simulink model "Lab3_Crazyflie_Task2_3"  (R2020a)
settings: Solver=FixedStepAuto  StartTime=0.0  StopTime=inf  MaxStep=0.1  RelTol=1e-3  EnableMultiTasking=on
PreLoadFcn:
  | % load parameters of the default quadrotor
  | disp('Quadrotor parameters loaded by PreLoadFcn')
  | mdl_quadrotor
values from neighbouring files (symbols this model uses):
  xx = via(:,1)    [Lab3_trajectories.m]
  yawyaw = 0 .* via(:,1)    [Lab3_trajectories.m]
  yy = via(:,2)    [Lab3_trajectories.m]
  zz = via(:,3) + 1    [Lab3_trajectories.m]
undefined symbols (not defined in the file or in its folder): angdiff, Pitch, Roll, rot2, Thrust, YawRate
libraries: simulink x7, robotlib x3
settings Model: Creator=corkep  LastModifiedBy=Pablo
settings DataIOCC: LimitDataPoints=on  ReturnWorkspaceOutputs=off
settings OptimizationCC: EnhancedBackFolding=on  PassReuseOutputArgsAs=Individual arguments  ExpressionDepthLimit=2147483647  ZeroExternalMemoryAtStartup=off  ZeroInternalMemoryAtStartup=off  MaxStackSize=64  OptimizeBlockOrder=speed  DifferentSizesBufferReuse=on  OptimizationCustomize=off  EfficientTunableParamExpr=on
settings DebuggingCC: UnderspecifiedInitializationDetection=Classic  MergeDetectMultiDrivingBlocksExec=none  SolverPrmCheckMsg=warning  ParameterTunabilityLossMsg=error  AllowSymbolicDim=off  StateNameClashWarn=warning  SFUnexpectedBacktrackingDiag=warning  SFNoUnconditionalDefaultTransitionDiag=warning  SFExecutionAtInitializationDiag=none  ArithmeticOperatorsInVariantConditions=warning
settings HardwareCC: ProdBitPerPointer=32  ProdBitPerSizeT=32  ProdBitPerPtrDiffT=32  ProdLargestAtomicFloat=None  ProdIntDivRoundTo=Undefined  ProdEndianess=Unspecified  ProdWordSize=32  ProdHWDeviceType=Generic->Unspecified (assume 32-bit Generic)  UseEmbeddedCoderFeatures=off
settings ModelReferenceCC: PropagateSignalLabelsOutOfModel=off
settings SFSimCC: SimUseLocalCustomCode=off  MATLABDynamicMemAlloc=off  CustomCodeUndefinedFunction=UseInterfaceOnly
settings RTWCC: SystemTargetFile=ert.tlc  HardwareBoard=Robot Operating System (ROS)  TemplateMakefile=ert_default_tmf  RTWUseLocalCustomCode=off  Toolchain=Catkin  TargetLang=C++
settings CodeAppCC: ForceParamTrailComments=on  IgnoreCustomStorageClasses=off  OperatorAnnotations=on  SimulinkDataObjDesc=on  SFDataObjDesc=on  InsertBlockDesc=on
settings ERTTargetCC: SupportNonInlinedSFcns=on
settings ConfigComp: CovMetricSettings=dw  CovHtmlReporting=on  CovSaveCumulativeToWorkspaceVar=on  CovSaveSingleToWorkspaceVar=on  CovExternalEMLEnable=off  CovSFcnEnable=off

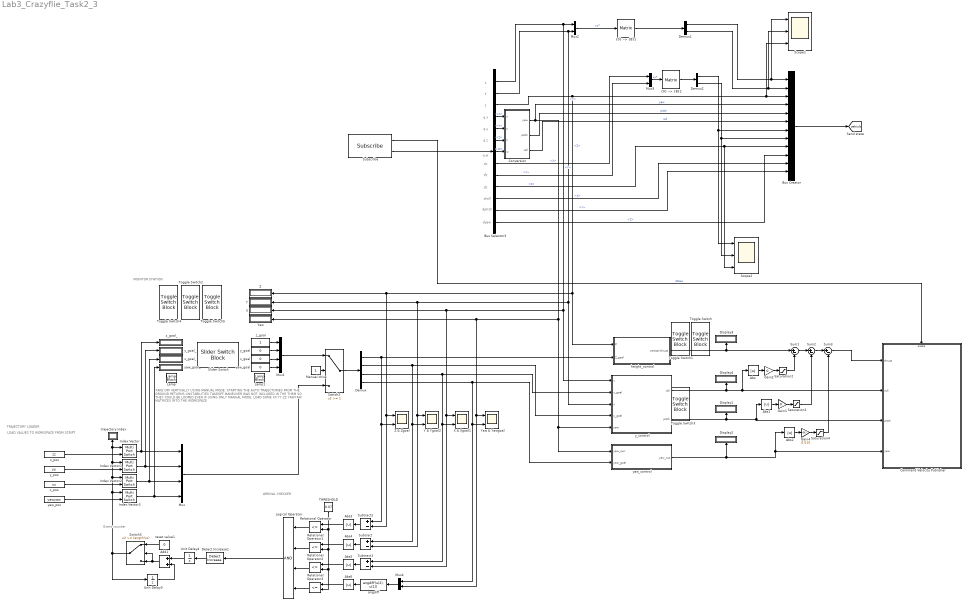
== system Lab3_Crazyflie_Task2_3 ==
  note: TAKE OFF VERTICALLY USING MANUAL MODE:
      | STARTING THE AUTO TRAJECTORIES FROM THE GROUND RETURNS UNSTABILITIES
      | TAKEOFF MANEUVER WAS NOT INCLUDED IN THE THEM SO THEY COULD BE LOOPED
      | EVEN IF USING ONLY MANUAL MODE, LOAD SOME XX YY ZZ YAWYAW MATRICES INTO THE WORKSPACE
  note: MONITOR STATION
  note: ARRIVAL CHECKER
  note: TRAJECTORY LOADER
  note: dyaw
  note: dpitch
  note: droll
  note: dz
  note: dy
  note: dx
  note: x
  note: y
  note: z
  note: q.x
  note: q.y
  note: q.z
  note: q.w
  note: LOAD VALUES TO WORKSPACE
      | FROM SCRIPT
  note: Event counter
  Abs{,1..6} (7 alike) : Abs
  Add1 : Sum
  Bus Creator : BusCreator  Inputs=12
  Bus Selector3 : BusSelector  OutputSignals=Pose.Pose.Position.X,Pose.Pose.Position.Y,Pose.Pose.Position.Z,Pose.Pose.Orientation.X,Pose.Pose.Orientation.Y,Pose.Pose.Orientation.Z,Pose.Pose.Orientation.W,Twist.Twist.Linear.X,Twist.Twist.Linear.Y,Twist.Twist.Linear.Z,Twist.Twist.Angular.X,Twist.Twist.Angular.Y,Twist.Twist.Angular.Z
  Command Velocity Publisher : Subsystem
  Conversion : MATLAB Function  TreatAsAtomicUnit=on
  Demux : Demux
  Demux1 : Demux  Outputs=2
  Demux2 : Demux  Outputs=2
  Detect Increase1 : simulink/Logic and Bit Operations/Detect Increase  vinit=0.0  OutDataTypeStr=boolean
  Display{1..4} (4 alike) : Display
  Gain1 : Gain  Gain=0
  Gain2 : Gain  Gain=0
  Gain4 : Gain  Gain=0.015
  Index Vector{,1..3} (4 alike) : MultiPortSwitch  DataPortOrder=Zero-based contiguous  Inputs=1  zeroidx=on
  Lamp : LampBlock
  Lamp1 : LampBlock
  Logical Operator : Logic  Inputs=4  AllPortsSameDT=off  OutDataTypeStr=boolean
  Manual drive : Constant
  Mux : Mux
  Mux1 : Mux
  Mux2 : Mux  Inputs=2
  Mux3 : Mux  Inputs=2
  Mux4 : Mux  Inputs=2
  Relational Operator{,1..3} (4 alike) : RelationalOperator  Operator=<=  OutDataTypeStr=boolean  RndMeth=Simplest
  Saturation1 : Saturate  LowerLimit=0
  Saturation2 : Saturate  LowerLimit=0
  Saturation4 : Saturate  LowerLimit=0
  Scope1 : Scope  NumInputPorts=3
  Scope2 : Scope  NumInputPorts=3
  Slider Switch : SliderSwitchBlock
      settings: Values={{'Auto', 'Manual'}, [0 1]}
  Subscribe : robotlib/Subscribe  topicSource=Select from ROS network  topic=/crazyflie2/ground_truth/odometry  messageType=nav_msgs/Odometry  sampleTime=-1  messageQueueLength=51
  Subtract : Sum  Inputs=+-
  Subtract1 : Sum  Inputs=+-
  Subtract2 : Sum  Inputs=+-
  Sum1 : Sum  Inputs=|+-
  Sum2 : Sum  Inputs=|+-
  Sum3 : Sum  Inputs=|+-
  Switch2 : Switch  Threshold=1
  Switch3 : Switch  Threshold=length(xx)
  THRESHOLD : Constant  Value=0.07
  Toggle Switch{,1..5} (6 alike) : ToggleSwitchBlock
      settings: Values={{'Off', 'On'}, [0 1]}
  Unit Delay3 : UnitDelay  SampleTime=-1  HasFrameUpgradeWarning=on
  Unit Delay4 : UnitDelay  SampleTime=-1  HasFrameUpgradeWarning=on
  X : Display
  X & Xgoal1 : Scope  NumInputPorts=2
  Y : Display
  Y & Ygoal2 : Scope  NumInputPorts=2
  Yaw : Display
  Yaw & Yawgoal : Scope  NumInputPorts=2
  Z : Display
  Z & Zgoal : Scope  NumInputPorts=2
  angdiff : MATLABFcn  MATLABFcn=angdiff(u(2), u(1))  OutputDimensions=1  Output1D=off
  height_control : Subsystem
  reset value1 : Constant  Value=0  VectorParams1D=off
  trajectory index : Display
  x_goal : Constant  Value=0
  x_goal_ : Display
  x_pos : Constant  Value=xx  VectorParams1D=off
  y_control : Subsystem
  y_goal : Constant  Value=0
  y_goal_ : Display
  y_pos : Constant  Value=yy  VectorParams1D=off
  yaw_control : Subsystem
  yaw_goal : Constant  Value=0
  yaw_goal_ : Display
  yaw_pos : Constant  Value=yawyaw  VectorParams1D=off
  z_goal : Constant
  z_goal_ : Display
  z_pos : Constant  Value=zz  VectorParams1D=off
  "{0} --> {B}1" : Product  Inputs=1  Multiplication=Matrix(*)  RndMeth=Zero
  "{0} --> {B}2" : Product  Inputs=1  Multiplication=Matrix(*)  RndMeth=Zero
  tag scope: vehicle=global
  wires:
  Bus Selector3/11 -> Bus Creator/11  "<X>"
  Bus Selector3/13 -> Bus Creator/10  "<Z>"
  Conversion/1(yaw) -> Bus Creator/4, yaw_control/1(yaw_curr), y_control/5(yaw), Yaw/1, Mux4/2, Yaw & Yawgoal/1  "yaw"
  Bus Selector3/10 -> Bus Creator/9, Scope2/3  "<Z>"
  Bus Selector3/9 -> Mux3/2  "<Y>"
  Bus Selector3/8 -> Mux3/1  "<X>"
  Conversion/2(pitch) -> Bus Creator/5  "pitch"
  Bus Selector3/3 -> Scope1/3, Bus Creator/3, height_control/1(Z), Subtract2/2, Z & Zgoal/1, Z/1  "<Z>"
  Bus Creator/1 -> [vehicle]
  Bus Selector3/12 -> Bus Creator/12  "<Y>"
  Conversion/3(roll) -> Bus Creator/6  "roll"
  Subscribe/2 -> Bus Selector3/1
  Bus Selector3/4 -> Conversion/1(x)  "<X>"
  Bus Selector3/5 -> Conversion/2(y)  "<Y>"
  Bus Selector3/6 -> Conversion/3(z)  "<Z>"
  Bus Selector3/7 -> Conversion/4(w)  "<W>"
  Subscribe/1 -> Command Velocity Publisher/Enable  "IsNew"
  Mux2/1 -> "{0} --> {B}1"/1  "xy*"
  "{0} --> {B}1"/1 -> Demux1/1
  "{0} --> {B}2"/1 -> Demux2/1
  Mux3/1 -> "{0} --> {B}2"/1  "xy*"
  Demux1/1 -> Bus Creator/1, Scope1/1
  Demux1/2 -> Bus Creator/2, Scope1/2
  Bus Selector3/1 -> Mux2/1, y_control/1(x), Subtract1/2, X & Xgoal1/1, X/1  "<X>"
  Demux2/1 -> Bus Creator/7, Scope2/1
  Demux2/2 -> Bus Creator/8, Scope2/2
  height_control/1(vertical thrust) -> Display3/1, Sum1/1
  Demux/1 -> Subtract2/1, Z & Zgoal/2, height_control/2(Z_goal)
  Bus Selector3/2 -> y_control/3(y), Subtract/2, Y & Ygoal2/1, Y/1, Mux2/2  "<Y>"
  Demux/3 -> X & Xgoal1/2, Subtract1/1, y_control/2(x_goal)
  Demux/4 -> Mux4/1, Yaw & Yawgoal/2, yaw_control/2(yaw_goal)
  Demux/2 -> Subtract/1, Y & Ygoal2/2, y_control/4(y_goal)
  Sum1/1 -> Sum2/1
  Sum2/1 -> Sum3/1
  Gain2/1 -> Saturation2/1
  Abs/1 -> Gain2/1
  Abs1/1 -> Gain1/1
  Gain1/1 -> Saturation1/1
  Saturation2/1 -> Sum1/2
  Saturation1/1 -> Sum2/2
  Abs2/1 -> Gain4/1
  Gain4/1 -> Saturation4/1
  Saturation4/1 -> Sum3/2
  z_pos/1 -> Index Vector/2
  y_pos/1 -> Index Vector1/2
  Index Vector2/1 -> Mux/3, x_goal_/1
  x_pos/1 -> Index Vector2/2
  Index Vector/1 -> Mux/1, z_goal_/1
  Index Vector1/1 -> Mux/2, y_goal_/1
  Switch3/1 -> Unit Delay3/1, trajectory index/1, Index Vector/1, Index Vector1/1, Index Vector2/1, Index Vector3/1
  yaw_pos/1 -> Index Vector3/2
  Index Vector3/1 -> yaw_goal_/1, Mux/4
  Mux/1 -> Switch2/3
  z_goal/1 -> Mux1/1
  y_goal/1 -> Mux1/2
  x_goal/1 -> Mux1/3
  yaw_goal/1 -> Mux1/4
  Mux1/1 -> Switch2/1
  Switch2/1 -> Demux/1
  Manual drive/1 -> Switch2/2
  Add1/1 -> Switch3/2, Switch3/3
  Unit Delay3/1 -> Add1/2
  reset value1/1 -> Switch3/1
  Detect Increase1/1 -> Unit Delay4/1
  Unit Delay4/1 -> Add1/1
  Logical Operator/1 -> Detect Increase1/1
  Mux4/1 -> angdiff/1
  Subtract2/1 -> Abs3/1
  Subtract/1 -> Abs4/1
  Subtract1/1 -> Abs5/1
  angdiff/1 -> Abs6/1
  Abs3/1 -> Relational Operator/1
  Abs4/1 -> Relational Operator1/1
  Abs5/1 -> Relational Operator2/1
  Abs6/1 -> Relational Operator3/1
  THRESHOLD/1 -> Relational Operator/2, Relational Operator1/2, Relational Operator2/2, Relational Operator3/2
  Relational Operator/1 -> Logical Operator/1
  Relational Operator1/1 -> Logical Operator/2
  Relational Operator2/1 -> Logical Operator/3
  Relational Operator3/1 -> Logical Operator/4
  Sum3/1 -> Command Velocity Publisher/1(thrust)
  y_control/1(roll) -> Display4/1, Abs/1, Command Velocity Publisher/2(roll)
  y_control/2(pitch) -> Display1/1, Abs1/1, Command Velocity Publisher/3(pitch)
  yaw_control/1(yaw_out) -> Display2/1, Command Velocity Publisher/4(yaw), Abs2/1

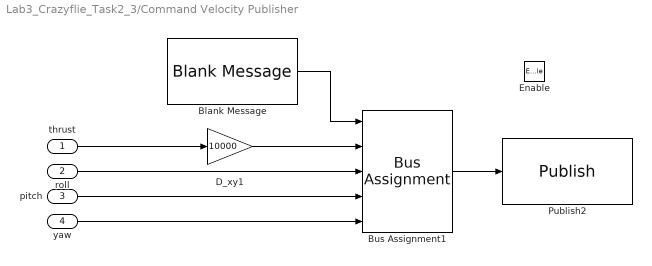
== system Lab3_Crazyflie_Task2_3/Command Velocity Publisher ==
  thrust : Inport
  roll : Inport  Port=2
  pitch : Inport  Port=3
  yaw : Inport  Port=4
  Enable : EnablePort
  Blank Message : robotlib/Blank Message  messageClass=Message  entityType=mav_msgs/RollPitchYawrateThrustCrazyflie  messageType=mav_msgs/RollPitchYawrateThrustCrazyflie  SampleTime=inf
  Bus Assignment1 : BusAssignment  DialogController=Simulink.DDGSource_BusAssignment  AssignedSignals=Thrust,Roll,Pitch,YawRate
  D_xy1 : Gain  Gain=10000
  Publish2 : robotlib/Publish  topicSource=Select from ROS network  topic=/crazyflie2/command/roll_pitch_yawrate_thrust  messageType=mav_msgs/RollPitchYawrateThrustCrazyflie  messageQueueLength=105
  wires:
  Blank Message/1 -> Bus Assignment1/1
  Bus Assignment1/1 -> Publish2/1
  thrust/1 -> D_xy1/1
  roll/1 -> Bus Assignment1/3
  pitch/1 -> Bus Assignment1/4
  yaw/1 -> Bus Assignment1/5
  D_xy1/1 -> Bus Assignment1/2

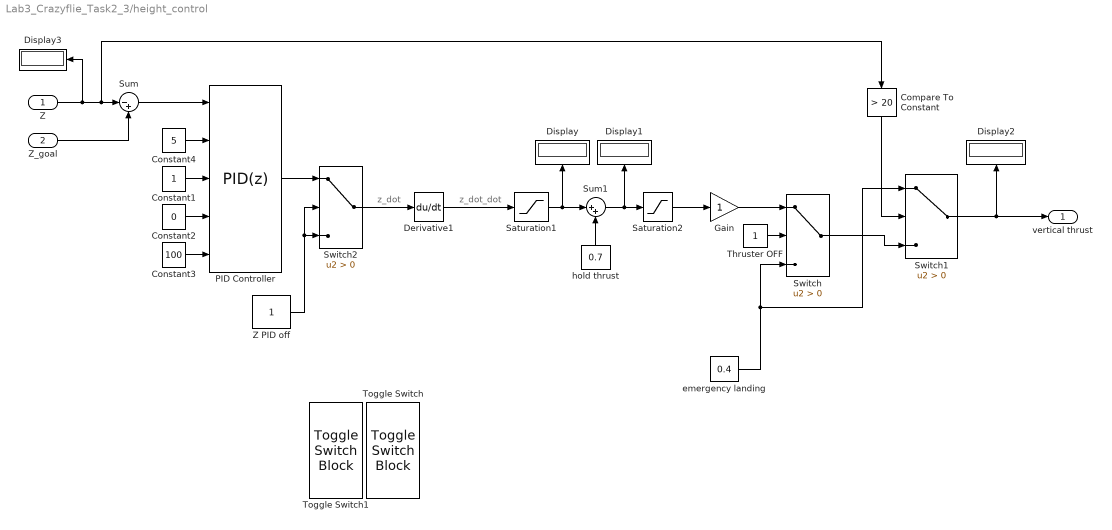
== system Lab3_Crazyflie_Task2_3/height_control ==
  note: z_dot
  note: z_dot_dot
  Z : Inport
  Z_goal : Inport  Port=2
  Compare To Constant : simulink/Logic and Bit Operations/Compare To Constant  relop=>  const=20  OutDataTypeStr=boolean
  Constant1 : Constant
  Constant2 : Constant  Value=0
  Constant3 : Constant  Value=100
  Constant4 : Constant  Value=5
  Derivative1 : Derivative
  Display{,1..3} (4 alike) : Display
  Gain : Gain
  PID Controller : simulink/Continuous/PID Controller  Controller=PID  Form=Parallel  TimeDomain=Discrete-time  UseExternalTs=off  SampleTime=-1  IntegratorMethod=Forward Euler  FilterMethod=Forward Euler  ControllerParametersSource=external  P=1  I=0  D=0  UseFilter=on  N=1000  TunerSelectOption=Transfer Function Based (PID Tuner App)  InitialConditionSource=internal  InitialConditionForIntegrator=0  InitialConditionForFilter=0  DifferentiatorICPrevScaledInput=0  ExternalReset=none  TrackingMode=off  Kt=1  LimitOutput=off  UpperSaturationLimit=inf  LowerSaturationLimit=-inf  LinearizeAsGain=on  AntiWindupMode=none  Kb=1  POutMin=[]  POutMax=[]  IOutMin=[]  IOutMax=[]  DOutMin=[]  DOutMax=[]  NOutMin=[]  NOutMax=[]  SumOutMin=[]  SumOutMax=[]  SaturationOutMin=[]  SaturationOutMax=[]  PParamMin=[]  PParamMax=[]  IParamMin=[]  IParamMax=[]  DParamMin=[]  DParamMax=[]  NParamMin=[]  NParamMax=[]  KbParamMin=[]  KbParamMax=[]  KtParamMin=[]  KtParamMax=[]  KbOutMin=[]  KbOutMax=[]  KtOutMin=[]  KtOutMax=[]  IntegratorOutMin=[]  IntegratorOutMax=[]  FilterOutMin=[]  FilterOutMax=[]  SumI1OutMin=[]  SumI1OutMax=[]  SumI2OutMin=[]  SumI2OutMax=[]  SumI3OutMin=[]  SumI3OutMax=[]  SumI4OutMin=[]  SumI4OutMax=[]  SumDOutMin=[]  SumDOutMax=[]  DifferentiatorOutMin=[]  DifferentiatorOutMax=[]  FilterDiffOutCoefMin=[]  FilterDiffOutCoefMax=[]  ReciprocalOutMin=[]  ReciprocalOutMax=[]  SumDenOutMin=[]  SumDenOutMax=[]  SumNumOutMin=[]  SumNumOutMax=[]  DivideOutMin=[]  DivideOutMax=[]  UdiffTsProdOutMin=[]  UdiffTsProdOutMax=[]  NTsProdOutMin=[]  NTsProdOutMax=[]  UintegralTsProdOutMin=[]  UintegralTsProdOutMax=[]  UngainTsProdOutMin=[]  UngainTsProdOutMax=[]  IntegratorContinuousStateAttributes=''  IntegratorStateMustResolveToSignalObject=off  IntegratorRTWStateStorageClass=Auto  FilterContinuousStateAttributes=''  FilterStateMustResolveToSignalObject=off  FilterRTWStateStorageClass=Auto  ParallelPVariant=ExternalParameters  IdealPVariant=Disabled  IVariant=ExternalParameters  DVariant=ExternalParameters  IntegratorVariant=Discrete  SatVariant=Disabled  AWVariant=Passthrough  PCopyVariant=Disabled  TRVariant=Disabled  FdbkBlocksVariant=Forward  IdealPFdbkVariant=Disabled  SatFdbkVariant=Disabled  DerivativeFilterVariant=ForwardEulerFilter  NVariant=ExternalParameters  NCopyVariant=Disabled  FilterICVariant=InternalICsFilter  IntegratorICVariant=InternalICs  ExternalResetVariant=Disabled  TRSumVariant=Passthrough  SumFdbkVariant=Disabled  SumVariant=Sum_PID  TsampFilterVariant=InternalTs  TsampNgainVariant=Passthrough  TsampIntegralVariant=Passthrough
  Saturation1 : Saturate  UpperLimit=99  LowerLimit=-99
  Saturation2 : Saturate  UpperLimit=1  LowerLimit=0
  Sum : Sum  Inputs=|-+
  Sum1 : Sum  Inputs=|++
  Switch : Switch  Criteria=u2 > Threshold
  Switch1 : Switch  Criteria=u2 > Threshold
  Switch2 : Switch  Criteria=u2 > Threshold
  Thruster OFF : Constant
  Toggle Switch : ToggleSwitchBlock
      settings: Values={{'Off', 'On'}, [0 1]}
  Toggle Switch1 : ToggleSwitchBlock
      settings: Values={{'Off', 'On'}, [0 1]}
  Z PID off : Constant
  emergency landing : Constant  Value=0.4
  hold thrust : Constant  Value=0.7
  vertical thrust : Outport
  wires:
  Z/1 -> Compare To Constant/1, Sum/1, Display3/1
  Constant4/1 -> PID Controller/2
  Constant1/1 -> PID Controller/3
  Constant2/1 -> PID Controller/4
  Constant3/1 -> PID Controller/5
  hold thrust/1 -> Sum1/2
  Saturation1/1 -> Sum1/1, Display/1
  Sum/1 -> PID Controller/1
  Thruster OFF/1 -> Switch/2
  Sum1/1 -> Saturation2/1, Display1/1
  Compare To Constant/1 -> Switch1/2
  emergency landing/1 -> Switch/3, Switch1/1
  Switch/1 -> Switch1/3
  Switch1/1 -> vertical thrust/1, Display2/1
  Z PID off/1 -> Switch2/2, Switch2/3
  PID Controller/1 -> Switch2/1
  Saturation2/1 -> Gain/1
  Switch2/1 -> Derivative1/1
  Derivative1/1 -> Saturation1/1
  Gain/1 -> Switch/1
  Z_goal/1 -> Sum/2

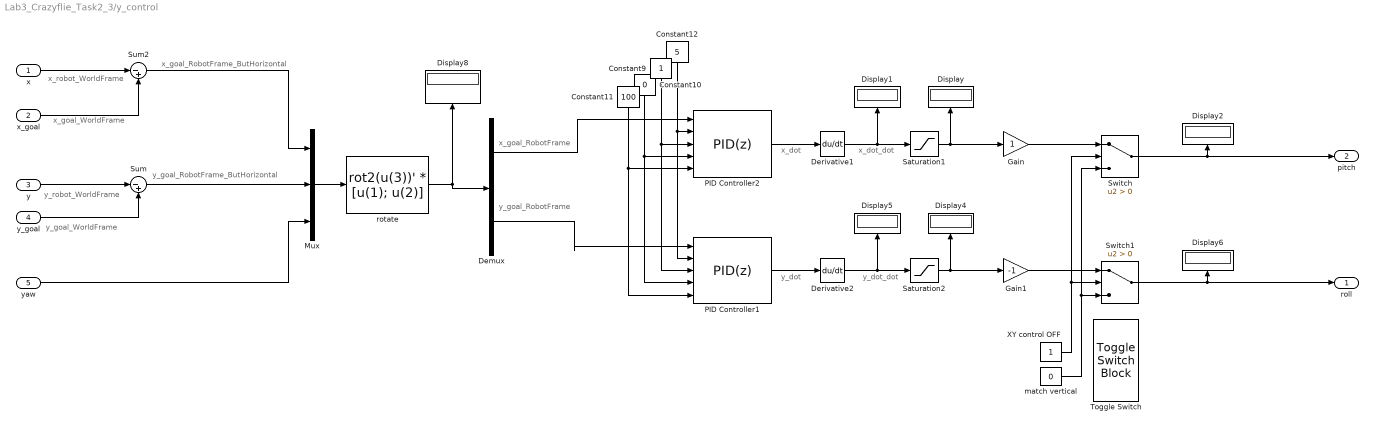
== system Lab3_Crazyflie_Task2_3/y_control ==
  note: y_goal_WorldFrame
  note: x_dot
  note: x_dot_dot
  note: y_robot_WorldFrame
  note: y_goal_RobotFrame_ButHorizontal
  note: y_dot
  note: y_dot_dot
  note: x_goal_RobotFrame_ButHorizontal
  note: x_goal_WorldFrame
  note: x_robot_WorldFrame
  note: x_goal_RobotFrame
  note: y_goal_RobotFrame
  x : Inport
  x_goal : Inport  Port=2
  y : Inport  Port=3
  y_goal : Inport  Port=4
  yaw : Inport  Port=5
  Constant10 : Constant  Value=0
  Constant11 : Constant  Value=100
  Constant12 : Constant  Value=5
  Constant9 : Constant
  Demux : Demux  Outputs=2
  Derivative1 : Derivative
  Derivative2 : Derivative
  Display{,1..2,4..6,8} (7 alike) : Display
  Gain : Gain
  Gain1 : Gain  Gain=-1
  Mux : Mux  Inputs=3
  PID Controller1 : simulink/Continuous/PID Controller  Controller=PID  Form=Parallel  TimeDomain=Discrete-time  UseExternalTs=off  SampleTime=-1  IntegratorMethod=Forward Euler  FilterMethod=Forward Euler  ControllerParametersSource=external  P=1  I=0  D=0  UseFilter=on  N=1000  TunerSelectOption=Transfer Function Based (PID Tuner App)  InitialConditionSource=internal  InitialConditionForIntegrator=0  InitialConditionForFilter=0  DifferentiatorICPrevScaledInput=0  ExternalReset=none  TrackingMode=off  Kt=1  LimitOutput=off  UpperSaturationLimit=inf  LowerSaturationLimit=-inf  LinearizeAsGain=on  AntiWindupMode=none  Kb=1  POutMin=[]  POutMax=[]  IOutMin=[]  IOutMax=[]  DOutMin=[]  DOutMax=[]  NOutMin=[]  NOutMax=[]  SumOutMin=[]  SumOutMax=[]  SaturationOutMin=[]  SaturationOutMax=[]  PParamMin=[]  PParamMax=[]  IParamMin=[]  IParamMax=[]  DParamMin=[]  DParamMax=[]  NParamMin=[]  NParamMax=[]  KbParamMin=[]  KbParamMax=[]  KtParamMin=[]  KtParamMax=[]  KbOutMin=[]  KbOutMax=[]  KtOutMin=[]  KtOutMax=[]  IntegratorOutMin=[]  IntegratorOutMax=[]  FilterOutMin=[]  FilterOutMax=[]  SumI1OutMin=[]  SumI1OutMax=[]  SumI2OutMin=[]  SumI2OutMax=[]  SumI3OutMin=[]  SumI3OutMax=[]  SumI4OutMin=[]  SumI4OutMax=[]  SumDOutMin=[]  SumDOutMax=[]  DifferentiatorOutMin=[]  DifferentiatorOutMax=[]  FilterDiffOutCoefMin=[]  FilterDiffOutCoefMax=[]  ReciprocalOutMin=[]  ReciprocalOutMax=[]  SumDenOutMin=[]  SumDenOutMax=[]  SumNumOutMin=[]  SumNumOutMax=[]  DivideOutMin=[]  DivideOutMax=[]  UdiffTsProdOutMin=[]  UdiffTsProdOutMax=[]  NTsProdOutMin=[]  NTsProdOutMax=[]  UintegralTsProdOutMin=[]  UintegralTsProdOutMax=[]  UngainTsProdOutMin=[]  UngainTsProdOutMax=[]  IntegratorContinuousStateAttributes=''  IntegratorStateMustResolveToSignalObject=off  IntegratorRTWStateStorageClass=Auto  FilterContinuousStateAttributes=''  FilterStateMustResolveToSignalObject=off  FilterRTWStateStorageClass=Auto  ParallelPVariant=ExternalParameters  IdealPVariant=Disabled  IVariant=ExternalParameters  DVariant=ExternalParameters  IntegratorVariant=Discrete  SatVariant=Disabled  AWVariant=Passthrough  PCopyVariant=Disabled  TRVariant=Disabled  FdbkBlocksVariant=Forward  IdealPFdbkVariant=Disabled  SatFdbkVariant=Disabled  DerivativeFilterVariant=ForwardEulerFilter  NVariant=ExternalParameters  NCopyVariant=Disabled  FilterICVariant=InternalICsFilter  IntegratorICVariant=InternalICs  ExternalResetVariant=Disabled  TRSumVariant=Passthrough  SumFdbkVariant=Disabled  SumVariant=Sum_PID  TsampFilterVariant=InternalTs  TsampNgainVariant=Passthrough  TsampIntegralVariant=Passthrough
  PID Controller2 : simulink/Continuous/PID Controller  Controller=PID  Form=Parallel  TimeDomain=Discrete-time  UseExternalTs=off  SampleTime=-1  IntegratorMethod=Forward Euler  FilterMethod=Forward Euler  ControllerParametersSource=external  P=1  I=0  D=0  UseFilter=on  N=1000  TunerSelectOption=Transfer Function Based (PID Tuner App)  InitialConditionSource=internal  InitialConditionForIntegrator=0  InitialConditionForFilter=0  DifferentiatorICPrevScaledInput=0  ExternalReset=none  TrackingMode=off  Kt=1  LimitOutput=off  UpperSaturationLimit=inf  LowerSaturationLimit=-inf  LinearizeAsGain=on  AntiWindupMode=none  Kb=1  POutMin=[]  POutMax=[]  IOutMin=[]  IOutMax=[]  DOutMin=[]  DOutMax=[]  NOutMin=[]  NOutMax=[]  SumOutMin=[]  SumOutMax=[]  SaturationOutMin=[]  SaturationOutMax=[]  PParamMin=[]  PParamMax=[]  IParamMin=[]  IParamMax=[]  DParamMin=[]  DParamMax=[]  NParamMin=[]  NParamMax=[]  KbParamMin=[]  KbParamMax=[]  KtParamMin=[]  KtParamMax=[]  KbOutMin=[]  KbOutMax=[]  KtOutMin=[]  KtOutMax=[]  IntegratorOutMin=[]  IntegratorOutMax=[]  FilterOutMin=[]  FilterOutMax=[]  SumI1OutMin=[]  SumI1OutMax=[]  SumI2OutMin=[]  SumI2OutMax=[]  SumI3OutMin=[]  SumI3OutMax=[]  SumI4OutMin=[]  SumI4OutMax=[]  SumDOutMin=[]  SumDOutMax=[]  DifferentiatorOutMin=[]  DifferentiatorOutMax=[]  FilterDiffOutCoefMin=[]  FilterDiffOutCoefMax=[]  ReciprocalOutMin=[]  ReciprocalOutMax=[]  SumDenOutMin=[]  SumDenOutMax=[]  SumNumOutMin=[]  SumNumOutMax=[]  DivideOutMin=[]  DivideOutMax=[]  UdiffTsProdOutMin=[]  UdiffTsProdOutMax=[]  NTsProdOutMin=[]  NTsProdOutMax=[]  UintegralTsProdOutMin=[]  UintegralTsProdOutMax=[]  UngainTsProdOutMin=[]  UngainTsProdOutMax=[]  IntegratorContinuousStateAttributes=''  IntegratorStateMustResolveToSignalObject=off  IntegratorRTWStateStorageClass=Auto  FilterContinuousStateAttributes=''  FilterStateMustResolveToSignalObject=off  FilterRTWStateStorageClass=Auto  ParallelPVariant=ExternalParameters  IdealPVariant=Disabled  IVariant=ExternalParameters  DVariant=ExternalParameters  IntegratorVariant=Discrete  SatVariant=Disabled  AWVariant=Passthrough  PCopyVariant=Disabled  TRVariant=Disabled  FdbkBlocksVariant=Forward  IdealPFdbkVariant=Disabled  SatFdbkVariant=Disabled  DerivativeFilterVariant=ForwardEulerFilter  NVariant=ExternalParameters  NCopyVariant=Disabled  FilterICVariant=InternalICsFilter  IntegratorICVariant=InternalICs  ExternalResetVariant=Disabled  TRSumVariant=Passthrough  SumFdbkVariant=Disabled  SumVariant=Sum_PID  TsampFilterVariant=InternalTs  TsampNgainVariant=Passthrough  TsampIntegralVariant=Passthrough
  Saturation1 : Saturate  UpperLimit=0.4  LowerLimit=-0.4
  Saturation2 : Saturate  UpperLimit=0.4  LowerLimit=-0.4
  Sum : Sum  Inputs=|-+
  Sum2 : Sum  Inputs=|-+
  Switch : Switch  Criteria=u2 > Threshold
  Switch1 : Switch  Criteria=u2 > Threshold
  Toggle Switch : ToggleSwitchBlock
      settings: Values={{'Off', 'On'}, [0 1]}
  XY control OFF : Constant
  match vertical : Constant  Value=0
  rotate : MATLABFcn  MATLABFcn=rot2(u(3))' * [u(1); u(2)]  OutputDimensions=[2 1]  Output1D=off
  roll : Outport
  pitch : Outport  Port=2
  wires:
  y/1 -> Sum/1
  y_goal/1 -> Sum/2
  Switch/1 -> Display2/1, pitch/1
  Saturation1/1 -> Gain/1, Display/1
  PID Controller2/1 -> Derivative1/1
  Derivative1/1 -> Saturation1/1, Display1/1
  Gain/1 -> Switch/1
  Saturation2/1 -> Gain1/1, Display4/1
  Switch1/1 -> roll/1, Display6/1
  Derivative2/1 -> Display5/1, Saturation2/1
  XY control OFF/1 -> Switch1/2, Switch/2
  Gain1/1 -> Switch1/1
  match vertical/1 -> Switch1/3, Switch/3
  x/1 -> Sum2/1
  x_goal/1 -> Sum2/2
  rotate/1 -> Display8/1, Demux/1
  Mux/1 -> rotate/1
  yaw/1 -> Mux/3
  Sum/1 -> Mux/2
  Sum2/1 -> Mux/1
  Demux/2 -> PID Controller1/1
  Constant9/1 -> PID Controller2/3, PID Controller1/3
  Constant12/1 -> PID Controller1/2, PID Controller2/2
  Constant10/1 -> PID Controller1/4, PID Controller2/4
  Constant11/1 -> PID Controller1/5, PID Controller2/5
  Demux/1 -> PID Controller2/1
  PID Controller1/1 -> Derivative2/1

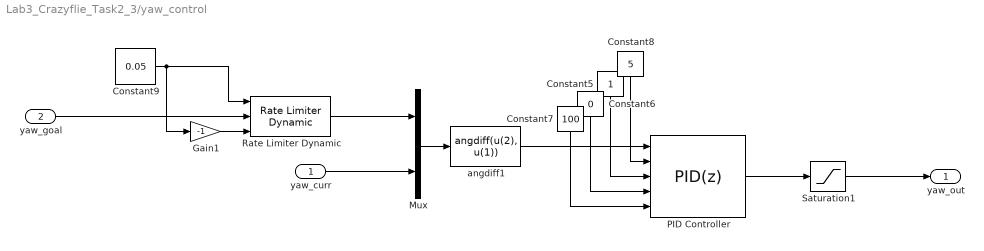
== system Lab3_Crazyflie_Task2_3/yaw_control ==
  yaw_curr : Inport
  yaw_goal : Inport  Port=2
  Constant5 : Constant
  Constant6 : Constant  Value=0
  Constant7 : Constant  Value=100
  Constant8 : Constant  Value=5
  Constant9 : Constant  Value=0.05
  Gain1 : Gain  Gain=-1
  Mux : Mux  Inputs=2
  PID Controller : simulink/Continuous/PID Controller  Controller=PID  Form=Parallel  TimeDomain=Discrete-time  UseExternalTs=off  SampleTime=-1  IntegratorMethod=Forward Euler  FilterMethod=Forward Euler  ControllerParametersSource=external  P=1  I=0  D=0  UseFilter=on  N=1000  TunerSelectOption=Transfer Function Based (PID Tuner App)  InitialConditionSource=internal  InitialConditionForIntegrator=0  InitialConditionForFilter=0  DifferentiatorICPrevScaledInput=0  ExternalReset=none  TrackingMode=off  Kt=1  LimitOutput=off  UpperSaturationLimit=inf  LowerSaturationLimit=-inf  LinearizeAsGain=on  AntiWindupMode=none  Kb=1  POutMin=[]  POutMax=[]  IOutMin=[]  IOutMax=[]  DOutMin=[]  DOutMax=[]  NOutMin=[]  NOutMax=[]  SumOutMin=[]  SumOutMax=[]  SaturationOutMin=[]  SaturationOutMax=[]  PParamMin=[]  PParamMax=[]  IParamMin=[]  IParamMax=[]  DParamMin=[]  DParamMax=[]  NParamMin=[]  NParamMax=[]  KbParamMin=[]  KbParamMax=[]  KtParamMin=[]  KtParamMax=[]  KbOutMin=[]  KbOutMax=[]  KtOutMin=[]  KtOutMax=[]  IntegratorOutMin=[]  IntegratorOutMax=[]  FilterOutMin=[]  FilterOutMax=[]  SumI1OutMin=[]  SumI1OutMax=[]  SumI2OutMin=[]  SumI2OutMax=[]  SumI3OutMin=[]  SumI3OutMax=[]  SumI4OutMin=[]  SumI4OutMax=[]  SumDOutMin=[]  SumDOutMax=[]  DifferentiatorOutMin=[]  DifferentiatorOutMax=[]  FilterDiffOutCoefMin=[]  FilterDiffOutCoefMax=[]  ReciprocalOutMin=[]  ReciprocalOutMax=[]  SumDenOutMin=[]  SumDenOutMax=[]  SumNumOutMin=[]  SumNumOutMax=[]  DivideOutMin=[]  DivideOutMax=[]  UdiffTsProdOutMin=[]  UdiffTsProdOutMax=[]  NTsProdOutMin=[]  NTsProdOutMax=[]  UintegralTsProdOutMin=[]  UintegralTsProdOutMax=[]  UngainTsProdOutMin=[]  UngainTsProdOutMax=[]  IntegratorContinuousStateAttributes=''  IntegratorStateMustResolveToSignalObject=off  IntegratorRTWStateStorageClass=Auto  FilterContinuousStateAttributes=''  FilterStateMustResolveToSignalObject=off  FilterRTWStateStorageClass=Auto  ParallelPVariant=ExternalParameters  IdealPVariant=Disabled  IVariant=ExternalParameters  DVariant=ExternalParameters  IntegratorVariant=Discrete  SatVariant=Disabled  AWVariant=Passthrough  PCopyVariant=Disabled  TRVariant=Disabled  FdbkBlocksVariant=Forward  IdealPFdbkVariant=Disabled  SatFdbkVariant=Disabled  DerivativeFilterVariant=ForwardEulerFilter  NVariant=ExternalParameters  NCopyVariant=Disabled  FilterICVariant=InternalICsFilter  IntegratorICVariant=InternalICs  ExternalResetVariant=Disabled  TRSumVariant=Passthrough  SumFdbkVariant=Disabled  SumVariant=Sum_PID  TsampFilterVariant=InternalTs  TsampNgainVariant=Passthrough  TsampIntegralVariant=Passthrough
  Rate Limiter Dynamic : simulink/Discontinuities/Rate Limiter Dynamic
  Saturation1 : Saturate  UpperLimit=20  LowerLimit=-20
  angdiff1 : MATLABFcn  MATLABFcn=angdiff(u(2), u(1))  OutputDimensions=1  Output1D=off
  yaw_out : Outport
  wires:
  Constant7/1 -> PID Controller/5
  Mux/1 -> angdiff1/1
  Constant9/1 -> Gain1/1, Rate Limiter Dynamic/1
  angdiff1/1 -> PID Controller/1
  Constant6/1 -> PID Controller/4
  Constant8/1 -> PID Controller/2
  Constant5/1 -> PID Controller/3
  PID Controller/1 -> Saturation1/1
  yaw_curr/1 -> Mux/2
  yaw_goal/1 -> Rate Limiter Dynamic/2
  Saturation1/1 -> yaw_out/1
  Gain1/1 -> Rate Limiter Dynamic/3
  Rate Limiter Dynamic/1 -> Mux/1

== matlab function Lab3_Crazyflie_Task2_3/Conversion ==
  data: yaw output; x input; y input; z input; w input; pitch output; roll output
function [yaw,pitch,roll]  = quat2eul(x,y,z,w)
%#codegen

% Convert the quaternion to a yaw angle (zyx euler angle)
eul = quat2eul([w,x,y,z]);
yaw = eul(1);
roll = eul(3);
pitch = eul(2);

end
